simulink model "DAS"  (R2012b)
settings: Solver=FixedStepDiscrete  StartTime=0.0  StopTime=inf  FixedStep=0.1  RelTol=1e-3
PreLoadFcn:
  | if exist('tl_preloadfcn','file'), tl_preloadfcn(gcs,101); end
PostLoadFcn:
  | if exist('tl_postloadfcn','file'), tl_postloadfcn(gcs,101); end
InitFcn:
  | if exist('tlds_init','file'), tlds_init(gcs); end
StartFcn:
  | if exist('tlds_start','file'), tlds_start(gcs); end
StopFcn:
  | if exist('tlds_stop','file'), tlds_stop(gcs); end
undefined symbols (not defined in the file): A, B, C, Dd, DEMO_FAS_Accusti_Threshold_Time, DEMO_FAS_BrakeBooster_Threshold, DEMO_FAS_CC_DELTA, DEMO_FAS_CC_Lvl2_Round, DEMO_FAS_CC_Min_Value, DEMO_FAS_Distance_Treshold_Far, DEMO_FAS_Distance_Treshold_Med, DEMO_FAS_Distance_Treshold_Near, DEMO_FAS_Distronic, DEMO_FAS_Emerg_Brake_Force1, DEMO_FAS_Emerg_Brake_Force2, DEMO_FAS_Emerg_Brake_Time1, DEMO_FAS_Emerg_Brake_Time2, DEMO_FAS_EmergencyBrake, DEMO_FAS_FollowToStop, DEMO_FAS_Limiter, DEMO_FAS_Limiter_DELTA, DEMO_FAS_Neg_Max_ms, DEMO_FAS_Opti_Threshold_Time, DEMO_FAS_Repeater, DEMO_FAS_Repeater_Time, DEMO_FAS_Signdetection, DEMO_FAS_Tempomat
(part 5 of 11)

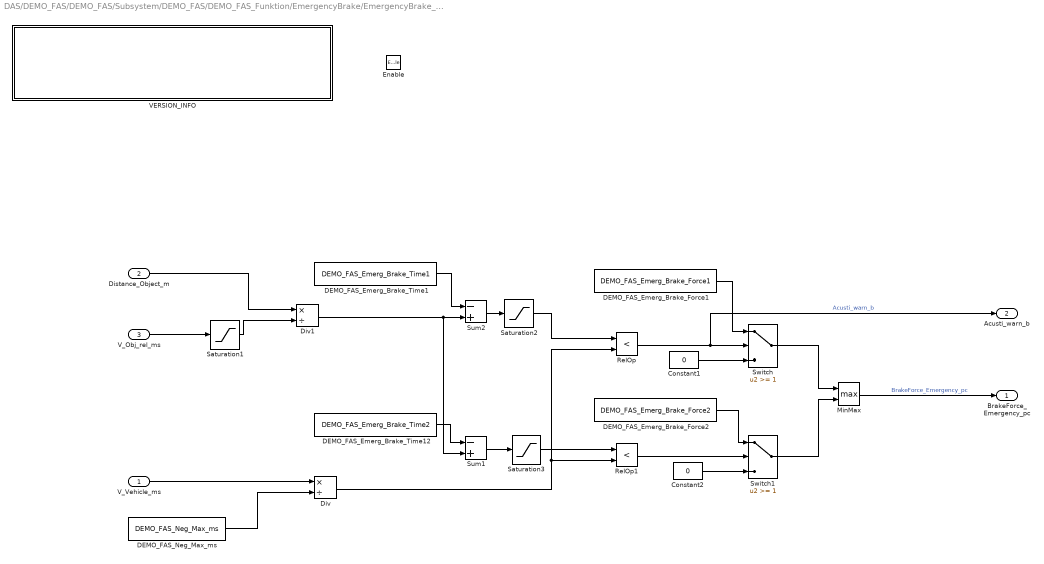
== system DAS/DEMO_FAS/DEMO_FAS/Subsystem/DEMO_FAS/DEMO_FAS_Funktion/EmergencyBrake/EmergencyBrake_Function ==
  V_Vehicle_ms : Inport
  Distance_Object_m : Inport  Port=2
  V_Obj_rel_ms : Inport  Port=3
  Enable : EnablePort  StatesWhenEnabling=reset
  Constant1 : Constant  Value=0  mask(TL_Constant){data={'date',735340.38498962962}}
      settings: CopyFcn=if exist('tl_reset_reviewflag') == 2, tl_reset_reviewflag(gcbh); end  DeleteFcn=if exist('delete_tlblock','file')==2,delete_tlblock(gcbh);end  NameChangeFcn=if exist('rename_tlblock','file')==2,rename_tlblock(gcbh);end  OpenFcn=if exist('tl_open_blockdlg','file')==2,tl_open_blockdlg(gcbh);else,open_system(gcbh,'parameter');end
      mask Help: eval(['if exist(''tl_online_help'',''file'') == 2, tl_online_help(''Topic'',''TL_Constant''),else, web([''jar:file:///'',matlabroot,''/help/toolbox/simulink/help.jar!/slref/' lower(get_param(gcbh,'Blocktype')) '.html''], ''-helpbrowser''),end'])
      mask Display: plot([-0.05, 1.05, NaN, -0.05, 1.05],[.01, .01, NaN, .99, .99])
  Constant2 : Constant  Value=0  mask(TL_Constant){data={'date',735340.38498962962}}
      settings: CopyFcn=if exist('tl_reset_reviewflag') == 2, tl_reset_reviewflag(gcbh); end  DeleteFcn=if exist('delete_tlblock','file')==2,delete_tlblock(gcbh);end  NameChangeFcn=if exist('rename_tlblock','file')==2,rename_tlblock(gcbh);end  OpenFcn=if exist('tl_open_blockdlg','file')==2,tl_open_blockdlg(gcbh);else,open_system(gcbh,'parameter');end
      mask Help: eval(['if exist(''tl_online_help'',''file'') == 2, tl_online_help(''Topic'',''TL_Constant''),else, web([''jar:file:///'',matlabroot,''/help/toolbox/simulink/help.jar!/slref/' lower(get_param(gcbh,'Blocktype')) '.html''], ''-helpbrowser''),end'])
      mask Display: plot([-0.05, 1.05, NaN, -0.05, 1.05],[.01, .01, NaN, .99, .99])
  DEMO_FAS_Emerg_Brake_Force1 : Constant  Description=|  Value=DEMO_FAS_Emerg_Brake_Force1  SampleTime=-1  mask(TL_Constant){data={'output',{'variable','DEMO_FAS/p/Components/DEMO_FAS_Emerg_Brake_Force1'},'date',735389.66854004632}}
      | Constant block of dSPACE TargetLink.
      | 
      | Output signal keeps the given constant value.
      settings: DeleteFcn=if exist('delete_tlblock','file')==2,delete_tlblock(gcbh);end  NameChangeFcn=if exist('rename_tlblock','file')==2,rename_tlblock(gcbh);end  OpenFcn=if exist('tl_open_blockdlg','file')==2,tl_open_blockdlg(gcbh);else,open_system(gcbh,'parameter');end
      mask Help: eval(['if exist(''tl_online_help'',''file'') == 2, tl_online_help(''Topic'',''TL_Constant''),else, web([''jar:file:///'',matlabroot,''/help/toolbox/simulink/help.jar!/slref/' lower(get_param(gcbh,'Blocktype')) '.html''], ''-helpbrowser''),end'])
      mask Display: plot([-0.05, 1.05, NaN, -0.05, 1.05],[.01, .01, NaN, .99, .99])
  DEMO_FAS_Emerg_Brake_Force2 : Constant  Description=|  Value=DEMO_FAS_Emerg_Brake_Force2  SampleTime=-1  mask(TL_Constant){data={'output',{'variable','DEMO_FAS/p/Components/DEMO_FAS_Emerg_Brake_Force2'},'date',735389.66865254624}}
      | Constant block of dSPACE TargetLink.
      | 
      | Output signal keeps the given constant value.
      settings: DeleteFcn=if exist('delete_tlblock','file')==2,delete_tlblock(gcbh);end  NameChangeFcn=if exist('rename_tlblock','file')==2,rename_tlblock(gcbh);end  OpenFcn=if exist('tl_open_blockdlg','file')==2,tl_open_blockdlg(gcbh);else,open_system(gcbh,'parameter');end
      mask Help: eval(['if exist(''tl_online_help'',''file'') == 2, tl_online_help(''Topic'',''TL_Constant''),else, web([''jar:file:///'',matlabroot,''/help/toolbox/simulink/help.jar!/slref/' lower(get_param(gcbh,'Blocktype')) '.html''], ''-helpbrowser''),end'])
      mask Display: plot([-0.05, 1.05, NaN, -0.05, 1.05],[.01, .01, NaN, .99, .99])
  DEMO_FAS_Emerg_Brake_Time1 : Constant  Description=|  Value=DEMO_FAS_Emerg_Brake_Time1  SampleTime=-1  mask(TL_Constant){data={'output',{'variable','DEMO_FAS/p/Components/DEMO_FAS_Emerg_Brake_Time1'},'date',735389.66832118051}}
      | Constant block of dSPACE TargetLink.
      | 
      | Output signal keeps the given constant value.
      settings: DeleteFcn=if exist('delete_tlblock','file')==2,delete_tlblock(gcbh);end  NameChangeFcn=if exist('rename_tlblock','file')==2,rename_tlblock(gcbh);end  OpenFcn=if exist('tl_open_blockdlg','file')==2,tl_open_blockdlg(gcbh);else,open_system(gcbh,'parameter');end
      mask Help: eval(['if exist(''tl_online_help'',''file'') == 2, tl_online_help(''Topic'',''TL_Constant''),else, web([''jar:file:///'',matlabroot,''/help/toolbox/simulink/help.jar!/slref/' lower(get_param(gcbh,'Blocktype')) '.html''], ''-helpbrowser''),end'])
      mask Display: plot([-0.05, 1.05, NaN, -0.05, 1.05],[.01, .01, NaN, .99, .99])
  DEMO_FAS_Emerg_Brake_Time12 : Constant  Description=|  Value=DEMO_FAS_Emerg_Brake_Time2  SampleTime=-1  mask(TL_Constant){data={'output',{'variable','DEMO_FAS/p/Components/DEMO_FAS_Emerg_Brake_Time2'},'date',735389.66844472219}}
      | Constant block of dSPACE TargetLink.
      | 
      | Output signal keeps the given constant value.
      settings: DeleteFcn=if exist('delete_tlblock','file')==2,delete_tlblock(gcbh);end  NameChangeFcn=if exist('rename_tlblock','file')==2,rename_tlblock(gcbh);end  OpenFcn=if exist('tl_open_blockdlg','file')==2,tl_open_blockdlg(gcbh);else,open_system(gcbh,'parameter');end
      mask Help: eval(['if exist(''tl_online_help'',''file'') == 2, tl_online_help(''Topic'',''TL_Constant''),else, web([''jar:file:///'',matlabroot,''/help/toolbox/simulink/help.jar!/slref/' lower(get_param(gcbh,'Blocktype')) '.html''], ''-helpbrowser''),end'])
      mask Display: plot([-0.05, 1.05, NaN, -0.05, 1.05],[.01, .01, NaN, .99, .99])
  DEMO_FAS_Neg_Max_ms : Constant  Description=|  Value=DEMO_FAS_Neg_Max_ms  SampleTime=-1  mask(TL_Constant){data={'output',{'variable','DEMO_FAS/p/Components/DEMO_FAS_Neg_Max_ms'},'date',735389.66875432874}}
      | Constant block of dSPACE TargetLink.
      | 
      | Output signal keeps the given constant value.
      settings: DeleteFcn=if exist('delete_tlblock','file')==2,delete_tlblock(gcbh);end  NameChangeFcn=if exist('rename_tlblock','file')==2,rename_tlblock(gcbh);end  OpenFcn=if exist('tl_open_blockdlg','file')==2,tl_open_blockdlg(gcbh);else,open_system(gcbh,'parameter');end
      mask Help: eval(['if exist(''tl_online_help'',''file'') == 2, tl_online_help(''Topic'',''TL_Constant''),else, web([''jar:file:///'',matlabroot,''/help/toolbox/simulink/help.jar!/slref/' lower(get_param(gcbh,'Blocktype')) '.html''], ''-helpbrowser''),end'])
      mask Display: plot([-0.05, 1.05, NaN, -0.05, 1.05],[.01, .01, NaN, .99, .99])
  Div : Product  Description=|  Inputs=*/  RndMeth=Zero  mask(TL_Product){data={'logdata',{'plotchannels',[]},'date',734383.73388777778}}
      | Product block of dSPACE TargetLink.
      | 
      | Output signal is equal to the product of the input signals. The input ports are specified according to conventions for Simulink Product blocks.
      settings: CopyFcn=if exist('tl_reset_reviewflag') == 2, tl_reset_reviewflag(gcbh); end  DeleteFcn=if exist('delete_tlblock','file')==2,delete_tlblock(gcbh);end  NameChangeFcn=if exist('rename_tlblock','file')==2,rename_tlblock(gcbh);end  OpenFcn=if exist('tl_open_blockdlg','file')==2,tl_open_blockdlg(gcbh);else,open_system(gcbh,'parameter');end
      mask Help: eval(['if exist(''tl_online_help'',''file'') == 2, tl_online_help(''Topic'',''TL_Product''),else, web([''jar:file:///'',matlabroot,''/help/toolbox/simulink/help.jar!/slref/' lower(get_param(gcbh,'Blocktype')) '.html''], ''-helpbrowser''),end'])
      mask Display: plot([-0.05, 1.05, NaN, -0.05, 1.05],[.01, .01, NaN, .99, .99])
  Div1 : Product  Description=|  Inputs=*/  RndMeth=Zero  mask(TL_Product){data={'logdata',{'plotchannels',[]},'date',734383.73388777778}}
      | Product block of dSPACE TargetLink.
      | 
      | Output signal is equal to the product of the input signals. The input ports are specified according to conventions for Simulink Product blocks.
      settings: CopyFcn=if exist('tl_reset_reviewflag') == 2, tl_reset_reviewflag(gcbh); end  DeleteFcn=if exist('delete_tlblock','file')==2,delete_tlblock(gcbh);end  NameChangeFcn=if exist('rename_tlblock','file')==2,rename_tlblock(gcbh);end  OpenFcn=if exist('tl_open_blockdlg','file')==2,tl_open_blockdlg(gcbh);else,open_system(gcbh,'parameter');end
      mask Help: eval(['if exist(''tl_online_help'',''file'') == 2, tl_online_help(''Topic'',''TL_Product''),else, web([''jar:file:///'',matlabroot,''/help/toolbox/simulink/help.jar!/slref/' lower(get_param(gcbh,'Blocktype')) '.html''], ''-helpbrowser''),end'])
      mask Display: plot([-0.05, 1.05, NaN, -0.05, 1.05],[.01, .01, NaN, .99, .99])
  MinMax : MinMax  Description=|  Function=max  Inputs=2  mask(TL_MinMax){data={'logdata',{'plotchannels',[]},'date',735383.52838311344}}
      | MinMax block of dSPACE TargetLink.
      | 
      | The MinMax block outputs either the minimum or the maximum element or elements of the input(s). If the block has one input port, the block outputs a scalar that is the minimum or maximum element of the input vector. If the block has more than one input port, the block performs an element-by-element comparison of the input vectors. Each element of the block output vector is the result of the comparison of the elements of the input vectors. The output of this block is equal to the greater or smaller input depending on the selected function.
      settings: CopyFcn=if exist('tl_reset_reviewflag') == 2, tl_reset_reviewflag(gcbh); end  DeleteFcn=if exist('delete_tlblock','file')==2,delete_tlblock(gcbh);end  NameChangeFcn=if exist('rename_tlblock','file')==2,rename_tlblock(gcbh);end  OpenFcn=if exist('tl_open_blockdlg','file')==2,tl_open_blockdlg(gcbh);else,open_system(gcbh,'parameter');end
      mask Help: eval(['if exist(''tl_online_help'',''file'') == 2, tl_online_help(''Topic'',''TL_MinMax''),else, web([''jar:file:///'',matlabroot,''/help/toolbox/simulink/help.jar!/slref/' lower(get_param(gcbh,'Blocktype')) '.html''], ''-helpbrowser''),end'])
      mask Display: plot([-0.05, 1.05, NaN, -0.05, 1.05],[.01, .01, NaN, .99, .99])
  RelOp : RelationalOperator  Description=|  Operator=<  mask(TL_RelationalOperator){data={'logdata',{'plotchannels',[]},'date',735389.55439398147}}
      | Relational operator block of dSPACE TargetLink.
      | 
      | This block performs a relational operation on its two inputs u1 and u2 and produces output according to the following table.
      | If the result is TRUE, the output is 1; if FALSE, it is 0.
      | 
      | Operator   Output
      |  ==        TRUE if u1 is equal to u2
      |  !=        TRUE if u1 is not equal to u2
      |  <         TRUE if u1 is less than u2
      |  <=        TRUE if u1 is less than or equal to u2
      |  >=        TRUE if u1 is greater than or equal to u2
      |  >         TRUE if u1 is greater than u2
      settings: DeleteFcn=if exist('delete_tlblock','file')==2,delete_tlblock(gcbh);end  NameChangeFcn=if exist('rename_tlblock','file')==2,rename_tlblock(gcbh);end  OpenFcn=if exist('tl_open_blockdlg','file')==2,tl_open_blockdlg(gcbh);else,open_system(gcbh,'parameter');end
      mask Help: eval(['if exist(''tl_online_help'',''file'') == 2, tl_online_help(''Topic'',''TL_RelationalOperator''),else, web([''jar:file:///'',matlabroot,''/help/toolbox/simulink/help.jar!/slref/' lower(get_param(gcbh,'Blocktype')) '.html''], ''-helpbrowser''),end'])
      mask Display: plot([-0.05, 1.05, NaN, -0.05, 1.05],[.01, .01, NaN, .99, .99])
  RelOp1 : RelationalOperator  Description=|  Operator=<  mask(TL_RelationalOperator){data={'logdata',{'plotchannels',[]},'date',735389.55444517359}}
      | Relational operator block of dSPACE TargetLink.
      | 
      | This block performs a relational operation on its two inputs u1 and u2 and produces output according to the following table.
      | If the result is TRUE, the output is 1; if FALSE, it is 0.
      | 
      | Operator   Output
      |  ==        TRUE if u1 is equal to u2
      |  !=        TRUE if u1 is not equal to u2
      |  <         TRUE if u1 is less than u2
      |  <=        TRUE if u1 is less than or equal to u2
      |  >=        TRUE if u1 is greater than or equal to u2
      |  >         TRUE if u1 is greater than u2
      settings: DeleteFcn=if exist('delete_tlblock','file')==2,delete_tlblock(gcbh);end  NameChangeFcn=if exist('rename_tlblock','file')==2,rename_tlblock(gcbh);end  OpenFcn=if exist('tl_open_blockdlg','file')==2,tl_open_blockdlg(gcbh);else,open_system(gcbh,'parameter');end
      mask Help: eval(['if exist(''tl_online_help'',''file'') == 2, tl_online_help(''Topic'',''TL_RelationalOperator''),else, web([''jar:file:///'',matlabroot,''/help/toolbox/simulink/help.jar!/slref/' lower(get_param(gcbh,'Blocktype')) '.html''], ''-helpbrowser''),end'])
      mask Display: plot([-0.05, 1.05, NaN, -0.05, 1.05],[.01, .01, NaN, .99, .99])
  Saturation1 : Saturate  UpperLimit=inf  LowerLimit=1  mask(TL_Saturate){data={'date',735389.55818375002}}
      settings: CopyFcn=if exist('tl_reset_reviewflag') == 2, tl_reset_reviewflag(gcbh); end  DeleteFcn=if exist('delete_tlblock','file')==2,delete_tlblock(gcbh);end  NameChangeFcn=if exist('rename_tlblock','file')==2,rename_tlblock(gcbh);end  OpenFcn=if exist('tl_open_blockdlg','file')==2,tl_open_blockdlg(gcbh);else,open_system(gcbh,'parameter');end
      mask Help: eval(['if exist(''tl_online_help'',''file'') == 2, tl_online_help(''Topic'',''TL_Saturate''),else, web([''jar:file:///'',matlabroot,''/help/toolbox/simulink/help.jar!/slref/' lower(get_param(gcbh,'Blocktype')) '.html''], ''-helpbrowser''),end'])
      mask Display: plot([-0.05, 1.05, NaN, -0.05, 1.05],[.01, .01, NaN, .99, .99])
  Saturation2 : Saturate  UpperLimit=inf  LowerLimit=1  mask(TL_Saturate){data={'date',735389.55818375002}}
      settings: CopyFcn=if exist('tl_reset_reviewflag') == 2, tl_reset_reviewflag(gcbh); end  DeleteFcn=if exist('delete_tlblock','file')==2,delete_tlblock(gcbh);end  NameChangeFcn=if exist('rename_tlblock','file')==2,rename_tlblock(gcbh);end  OpenFcn=if exist('tl_open_blockdlg','file')==2,tl_open_blockdlg(gcbh);else,open_system(gcbh,'parameter');end
      mask Help: eval(['if exist(''tl_online_help'',''file'') == 2, tl_online_help(''Topic'',''TL_Saturate''),else, web([''jar:file:///'',matlabroot,''/help/toolbox/simulink/help.jar!/slref/' lower(get_param(gcbh,'Blocktype')) '.html''], ''-helpbrowser''),end'])
      mask Display: plot([-0.05, 1.05, NaN, -0.05, 1.05],[.01, .01, NaN, .99, .99])
  Saturation3 : Saturate  UpperLimit=inf  LowerLimit=1  mask(TL_Saturate){data={'date',735389.55818375002}}
      settings: CopyFcn=if exist('tl_reset_reviewflag') == 2, tl_reset_reviewflag(gcbh); end  DeleteFcn=if exist('delete_tlblock','file')==2,delete_tlblock(gcbh);end  NameChangeFcn=if exist('rename_tlblock','file')==2,rename_tlblock(gcbh);end  OpenFcn=if exist('tl_open_blockdlg','file')==2,tl_open_blockdlg(gcbh);else,open_system(gcbh,'parameter');end
      mask Help: eval(['if exist(''tl_online_help'',''file'') == 2, tl_online_help(''Topic'',''TL_Saturate''),else, web([''jar:file:///'',matlabroot,''/help/toolbox/simulink/help.jar!/slref/' lower(get_param(gcbh,'Blocktype')) '.html''], ''-helpbrowser''),end'])
      mask Display: plot([-0.05, 1.05, NaN, -0.05, 1.05],[.01, .01, NaN, .99, .99])
  Sum1 : Sum  Description=|  Inputs=-+  mask(TL_Sum){data={'logdata',{'plotchannels',[]},'date',735383.47236888891}}
      | Sum block of dSPACE TargetLink.
      | 
      | Output signal is equal to the sum of the input signals.
      | The list of signs is specified according to conventions for Simulink Sum blocks.
      settings: CopyFcn=if exist('tl_reset_reviewflag') == 2, tl_reset_reviewflag(gcbh); end  DeleteFcn=if exist('delete_tlblock','file')==2,delete_tlblock(gcbh);end  NameChangeFcn=if exist('rename_tlblock','file')==2,rename_tlblock(gcbh);end  OpenFcn=if exist('tl_open_blockdlg','file')==2,tl_open_blockdlg(gcbh);else,open_system(gcbh,'parameter');end
      mask Help: eval(['if exist(''tl_online_help'',''file'') == 2, tl_online_help(''Topic'',''TL_Sum''),else, web([''jar:file:///'',matlabroot,''/help/toolbox/simulink/help.jar!/slref/' lower(get_param(gcbh,'Blocktype')) '.html''], ''-helpbrowser''),end'])
      mask Display: plot([-0.05, 1.05, NaN, -0.05, 1.05],[.01, .01, NaN, .99, .99])
  Sum2 : Sum  Description=|  Inputs=-+  mask(TL_Sum){data={'logdata',{'plotchannels',[]},'date',735383.47236888891}}
      | Sum block of dSPACE TargetLink.
      | 
      | Output signal is equal to the sum of the input signals.
      | The list of signs is specified according to conventions for Simulink Sum blocks.
      settings: CopyFcn=if exist('tl_reset_reviewflag') == 2, tl_reset_reviewflag(gcbh); end  DeleteFcn=if exist('delete_tlblock','file')==2,delete_tlblock(gcbh);end  NameChangeFcn=if exist('rename_tlblock','file')==2,rename_tlblock(gcbh);end  OpenFcn=if exist('tl_open_blockdlg','file')==2,tl_open_blockdlg(gcbh);else,open_system(gcbh,'parameter');end
      mask Help: eval(['if exist(''tl_online_help'',''file'') == 2, tl_online_help(''Topic'',''TL_Sum''),else, web([''jar:file:///'',matlabroot,''/help/toolbox/simulink/help.jar!/slref/' lower(get_param(gcbh,'Blocktype')) '.html''], ''-helpbrowser''),end'])
      mask Display: plot([-0.05, 1.05, NaN, -0.05, 1.05],[.01, .01, NaN, .99, .99])
  Switch : Switch  Threshold=1  mask(TL_Switch){data={'date',735389.55168915505}}
      settings: CopyFcn=if exist('tl_reset_reviewflag') == 2, tl_reset_reviewflag(gcbh); end  DeleteFcn=if exist('delete_tlblock','file')==2,delete_tlblock(gcbh);end  NameChangeFcn=if exist('rename_tlblock','file')==2,rename_tlblock(gcbh);end  OpenFcn=if exist('tl_open_blockdlg','file')==2,tl_open_blockdlg(gcbh);else,open_system(gcbh,'parameter');end
      mask Help: eval(['if exist(''tl_online_help'',''file'') == 2, tl_online_help(''Topic'',''TL_Switch''),else, web([''jar:file:///'',matlabroot,''/help/toolbox/simulink/help.jar!/slref/' lower(get_param(gcbh,'Blocktype')) '.html''], ''-helpbrowser''),end'])
      mask Display: plot([-0.05, 1.05, NaN, -0.05, 1.05],[.01, .01, NaN, .99, .99])
  Switch1 : Switch  Threshold=1  mask(TL_Switch){data={'date',735383.52020709496}}
      settings: CopyFcn=if exist('tl_reset_reviewflag') == 2, tl_reset_reviewflag(gcbh); end  DeleteFcn=if exist('delete_tlblock','file')==2,delete_tlblock(gcbh);end  NameChangeFcn=if exist('rename_tlblock','file')==2,rename_tlblock(gcbh);end  OpenFcn=if exist('tl_open_blockdlg','file')==2,tl_open_blockdlg(gcbh);else,open_system(gcbh,'parameter');end
      mask Help: eval(['if exist(''tl_online_help'',''file'') == 2, tl_online_help(''Topic'',''TL_Switch''),else, web([''jar:file:///'',matlabroot,''/help/toolbox/simulink/help.jar!/slref/' lower(get_param(gcbh,'Blocktype')) '.html''], ''-helpbrowser''),end'])
      mask Display: plot([-0.05, 1.05, NaN, -0.05, 1.05],[.01, .01, NaN, .99, .99])
  VERSION_INFO : Subsystem  mask(VERSION_INFO_BLOCK){versinfo_data=struct('modname','DEMO_FAS/DEMO_FAS_Funktion/EmergencyBrake/EmergencyBrake_Function','version','1.1.1','date','29-May-2013','author','YVEDUHR','modtype',3,'variant',0,'remark',{{'~'}},'copyright',['Daimler AG'],'SGMLdescr','','prefix','','pfx_act',0,'ntselect',3,'asize',0), versinfo_string=Model: DEMO_FAS/DEMO_FAS_Funktion/EmergencyBrake/EmergencyBrake_Function\nVersion: 1.1.1\nDate: 29-May-2013\nAuthor: YVEDUHR\nModule: INTERNAL\n\nAll copyrights by Daimler AG}
      mask prompts: versinfo_data "Mask Parameter 1"; versinfo_string "Mask Parameter 2"
      mask help:
      | This is a Version Info Subsystem (empty)
      | All version Information is stored in Parameter "versinfo_data" and displayed
      settings: OpenFcn=edit_subsys_info('init')
      mask Display: disp(versinfo_string);
  BrakeForce_Emergency_pc : Outport  InitialOutput=0
  Acusti_warn_b : Outport  Port=2  InitialOutput=0
  wires:
  V_Vehicle_ms/1 -> Div/1
  DEMO_FAS_Neg_Max_ms/1 -> Div/2
  Div/1 -> RelOp/2, RelOp1/2
  Distance_Object_m/1 -> Div1/1
  V_Obj_rel_ms/1 -> Saturation1/1
  DEMO_FAS_Emerg_Brake_Time1/1 -> Sum2/1
  DEMO_FAS_Emerg_Brake_Time12/1 -> Sum1/1
  Sum2/1 -> Saturation2/1
  Sum1/1 -> Saturation3/1
  RelOp/1 -> Acusti_warn_b/1, Switch/2  "Acusti_warn_b"
  DEMO_FAS_Emerg_Brake_Force1/1 -> Switch/1
  DEMO_FAS_Emerg_Brake_Force2/1 -> Switch1/1
  RelOp1/1 -> Switch1/2
  Constant1/1 -> Switch/3
  Constant2/1 -> Switch1/3
  Switch/1 -> MinMax/1
  Switch1/1 -> MinMax/2
  MinMax/1 -> BrakeForce_Emergency_pc/1  "BrakeForce_Emergency_pc"
  Div1/1 -> Sum1/2, Sum2/2
  Saturation1/1 -> Div1/2
  Saturation2/1 -> RelOp/1
  Saturation3/1 -> RelOp1/1

== system DAS/DEMO_FAS/DEMO_FAS/Subsystem/DEMO_FAS/DEMO_FAS_Funktion/EmergencyBrake/VERSION_INFO ==
  Copyright : Subsystem
      mask help: Copyright
      mask Display: disp('All copyrights by DaimlerChrysler');

== system DAS/DEMO_FAS/DEMO_FAS/Subsystem/DEMO_FAS/DEMO_FAS_Funktion/FAS_Input/VERSION_INFO ==
  Copyright : Subsystem
      mask help: Copyright
      mask Display: disp('All copyrights by DaimlerChrysler');

== system DAS/DEMO_FAS/DEMO_FAS/Subsystem/DEMO_FAS/DEMO_FAS_Funktion/FollowToStop/FollowToStop_Function ==
  V_Vehicle_kmh : Inport
  V_Obj_rel_kmh : Inport  Port=2
  Enable : EnablePort  StatesWhenEnabling=reset
  Chart : Stateflow chart  TreatAsAtomicUnit=on
  Sum : Sum  Description=|  Inputs=+-  mask(TL_Sum){data={'logdata',{'plotchannels',[]},'date',735388.57141554402}}
      | Sum block of dSPACE TargetLink.
      | 
      | Output signal is equal to the sum of the input signals.
      | The list of signs is specified according to conventions for Simulink Sum blocks.
      settings: CopyFcn=if exist('tl_reset_reviewflag') == 2, tl_reset_reviewflag(gcbh); end  DeleteFcn=if exist('delete_tlblock','file')==2,delete_tlblock(gcbh);end  NameChangeFcn=if exist('rename_tlblock','file')==2,rename_tlblock(gcbh);end  OpenFcn=if exist('tl_open_blockdlg','file')==2,tl_open_blockdlg(gcbh);else,open_system(gcbh,'parameter');end
      mask Help: eval(['if exist(''tl_online_help'',''file'') == 2, tl_online_help(''Topic'',''TL_Sum''),else, web([''jar:file:///'',matlabroot,''/help/toolbox/simulink/help.jar!/slref/' lower(get_param(gcbh,'Blocktype')) '.html''], ''-helpbrowser''),end'])
      mask Display: plot([-0.05, 1.05, NaN, -0.05, 1.05],[.01, .01, NaN, .99, .99])
  VERSION_INFO : Subsystem  mask(VERSION_INFO_BLOCK){versinfo_data=struct('modname','DEMO_FAS/DEMO_FAS_Funktion/FollowToStop/FollowToStop_Function','version','1.1.1','date','23-May-2013','author','YVEDUHR','modtype',3,'variant',0,'remark',{{'~'}},'copyright',['Daimler AG'],'SGMLdescr','','prefix','','pfx_act',0,'ntselect',3,'asize',0), versinfo_string=Model: DEMO_FAS/DEMO_FAS_Funktion/FollowToStop/FollowToStop_Function\nVersion: 1.1.1\nDate: 23-May-2013\nAuthor: YVEDUHR\nModule: INTERNAL\n\nAll copyrights by Daimler AG}
      mask prompts: versinfo_data "Mask Parameter 1"; versinfo_string "Mask Parameter 2"
      mask help:
      | This is a Version Info Subsystem (empty)
      | All version Information is stored in Parameter "versinfo_data" and displayed
      settings: OpenFcn=edit_subsys_info('init')
      mask Display: disp(versinfo_string);
  FTS_active_b : Outport
  FTS_Abstand_soll_m : Outport  Port=2
  wires:
  V_Obj_rel_kmh/1 -> Sum/2
  V_Vehicle_kmh/1 -> Sum/1
  Sum/1 -> Chart/1(V_Obj_kmh)  "V_Obj_kmh"
  Chart/1(FTS_active_b) -> FTS_active_b/1  "FTS_active_b"
  Chart/2(Abstand_soll_m) -> FTS_Abstand_soll_m/1  "FTS_Abstand_soll_m"

== system DAS/DEMO_FAS/DEMO_FAS/Subsystem/DEMO_FAS/DEMO_FAS_Funktion/FollowToStop/VERSION_INFO ==
  Copyright : Subsystem
      mask help: Copyright
      mask Display: disp('All copyrights by DaimlerChrysler');

== system DAS/DEMO_FAS/DEMO_FAS/Subsystem/DEMO_FAS/DEMO_FAS_Funktion/Limiter/Limiter_Function ==
  Limiter_b : Inport
  Accelaration_pedal_pc : Inport  Port=2
  V_Vehicle_kmh : Inport  Port=3
  LeverUp_stat : Inport  Port=4
  LeverDown_stat : Inport  Port=5
  V_Sign_kmh : Inport  Port=6
  Sign_b : Inport  Port=7
  Enable : EnablePort
  DEMO_FAS_Signdetection : Constant  Description=|  Value=DEMO_FAS_Signdetection  SampleTime=-1  mask(TL_Constant){data={'output',{'variable','DEMO_FAS/p/Components/DEMO_FAS_Signdetection'},'date',735441.46049939818}}
      | Constant block of dSPACE TargetLink.
      | 
      | Output signal keeps the given constant value.
      settings: DeleteFcn=if exist('delete_tlblock','file')==2,delete_tlblock(gcbh);end  NameChangeFcn=if exist('rename_tlblock','file')==2,rename_tlblock(gcbh);end  OpenFcn=if exist('tl_open_blockdlg','file')==2,tl_open_blockdlg(gcbh);else,open_system(gcbh,'parameter');end
      mask Help: eval(['if exist(''tl_online_help'',''file'') == 2, tl_online_help(''Topic'',''TL_Constant''),else, web([''jar:file:///'',matlabroot,''/help/toolbox/simulink/help.jar!/slref/' lower(get_param(gcbh,'Blocktype')) '.html''], ''-helpbrowser''),end'])
      mask Display: plot([-0.05, 1.05, NaN, -0.05, 1.05],[.01, .01, NaN, .99, .99])
  Limiter_Enabled : Subsystem
  Limiter_InitialSetValue : Subsystem  TreatAsAtomicUnit=on
  Limiter_SetValue : Subsystem
  Limiter_StartUpSetValue : Subsystem  TreatAsAtomicUnit=on
  Logical Operator : Logic  AllPortsSameDT=off  OutDataTypeStr=boolean  mask(TL_LogicalOperator){data={'date',735360.45292877313}}
      settings: DeleteFcn=if exist('delete_tlblock','file')==2,delete_tlblock(gcbh);end  NameChangeFcn=if exist('rename_tlblock','file')==2,rename_tlblock(gcbh);end  OpenFcn=if exist('tl_open_blockdlg','file')==2,tl_open_blockdlg(gcbh);else,open_system(gcbh,'parameter');end
      mask Help: eval(['if exist(''tl_online_help'',''file'') == 2, tl_online_help(''Topic'',''TL_LogicalOperator''),else, web([''jar:file:///'',matlabroot,''/help/toolbox/simulink/help.jar!/slref/' lower(get_param(gcbh,'Blocktype')) '.html''], ''-helpbrowser''),end'])
      mask Display: plot([-0.05, 1.05, NaN, -0.05, 1.05],[.01, .01, NaN, .99, .99])
  MinMax : MinMax  Inputs=2  mask(TL_MinMax){data={'date',735369.40750826395}}
      settings: CopyFcn=if exist('tl_reset_reviewflag') == 2, tl_reset_reviewflag(gcbh); end  DeleteFcn=if exist('delete_tlblock','file')==2,delete_tlblock(gcbh);end  NameChangeFcn=if exist('rename_tlblock','file')==2,rename_tlblock(gcbh);end  OpenFcn=if exist('tl_open_blockdlg','file')==2,tl_open_blockdlg(gcbh);else,open_system(gcbh,'parameter');end
      mask Help: eval(['if exist(''tl_online_help'',''file'') == 2, tl_online_help(''Topic'',''TL_MinMax''),else, web([''jar:file:///'',matlabroot,''/help/toolbox/simulink/help.jar!/slref/' lower(get_param(gcbh,'Blocktype')) '.html''], ''-helpbrowser''),end'])
      mask Display: plot([-0.05, 1.05, NaN, -0.05, 1.05],[.01, .01, NaN, .99, .99])
  Switch : Switch  Threshold=1  mask(TL_Switch){data={'date',735369.40809475689}}
      settings: CopyFcn=if exist('tl_reset_reviewflag') == 2, tl_reset_reviewflag(gcbh); end  DeleteFcn=if exist('delete_tlblock','file')==2,delete_tlblock(gcbh);end  NameChangeFcn=if exist('rename_tlblock','file')==2,rename_tlblock(gcbh);end  OpenFcn=if exist('tl_open_blockdlg','file')==2,tl_open_blockdlg(gcbh);else,open_system(gcbh,'parameter');end
      mask Help: eval(['if exist(''tl_online_help'',''file'') == 2, tl_online_help(''Topic'',''TL_Switch''),else, web([''jar:file:///'',matlabroot,''/help/toolbox/simulink/help.jar!/slref/' lower(get_param(gcbh,'Blocktype')) '.html''], ''-helpbrowser''),end'])
      mask Display: plot([-0.05, 1.05, NaN, -0.05, 1.05],[.01, .01, NaN, .99, .99])
  SysInit : Subsystem  mask(TLACT_SG_V200_SysInit){dT=-1, YName=}
      mask prompts: dT "Sample Time"; YName "Y OutName"
      mask help: An inital pulse is generated for for the first block evaluation.
      mask init:
      | % TL block lines
      | x1=[0 0 1 1 0];
      | y1=[1 0 0 1 1];
      | x2=[1 0];
      | y2=[.92 .92];
      | x3=[0 1];
      | y3=[.08 .08];
      | 
      | tl_act_sg_init_blk;
      mask Help:
      | <P><B>Function:</B></P>
      | <P>The block provides an initial pulse at the output on the first
      | evaluation of the block.<BR> This function can be used for system startup functions to
      | get defined states in the system.</P>
      | 
      | <P><B>In-/Outputs:</B></P>
      | <P><U>Output</U></P>
      | <P>The output shows TRUE at the first cycle, else it shows FALSE.</P>
      mask Display:
      | plot(x1,y1,x2,y2,x3,y3);
      | disp('SysInit');
  VERSION_INFO : Subsystem  mask(VERSION_INFO_BLOCK){versinfo_data=struct('modname','DEMO_FAS/DEMO_FAS_Funktion/Limiter/Limiter_Function','version','1.1.1','date','18-Apr-2013','author','YVEDUHR','modtype',3,'variant',0,'remark',{{'~'}},'copyright',['Daimler AG'],'SGMLdescr','','prefix','','pfx_act',0,'ntselect',3,'asize',0), versinfo_string=Model: DEMO_FAS/DEMO_FAS_Funktion/Limiter/Limiter_Function\nVersion: 1.1.1\nDate: 18-Apr-2013\nAuthor: YVEDUHR\nModule: INTERNAL\n\nAll copyrights by Daimler AG}
      mask prompts: versinfo_data "Mask Parameter 1"; versinfo_string "Mask Parameter 2"
      mask help:
      | This is a Version Info Subsystem (empty)
      | All version Information is stored in Parameter "versinfo_data" and displayed
      settings: OpenFcn=edit_subsys_info('init')
      mask Display: disp(versinfo_string);
  VMax_kmh : Outport
  Limiter_active_b : Outport  Port=2  InitialOutput=0
  wires:
  LeverDown_stat/1 -> Limiter_SetValue/2(LeverDown_stat)
  LeverUp_stat/1 -> Limiter_SetValue/1(LeverUp_stat)
  V_Vehicle_kmh/1 -> Limiter_InitialSetValue/1(V_Vehicle_kmh)
  Limiter_Enabled/1(VMax_kmh) -> MinMax/2, Switch/3
  Limiter_b/1 -> Limiter_InitialSetValue/Trigger, Limiter_SetValue/Enable, Limiter_Enabled/1(Limiter_b)
  Accelaration_pedal_pc/1 -> Limiter_Enabled/2(Accelaration_pedal_pc)
  Limiter_Enabled/2(Limiter_active_b) -> Limiter_active_b/1
  SysInit/1(y) -> Limiter_StartUpSetValue/Trigger
  Switch/1 -> VMax_kmh/1  "VMax_kmh"
  Sign_b/1 -> Logical Operator/1
  MinMax/1 -> Switch/1
  V_Sign_kmh/1 -> MinMax/1
  DEMO_FAS_Signdetection/1 -> Logical Operator/2
  Logical Operator/1 -> Switch/2

== system DAS/DEMO_FAS/DEMO_FAS/Subsystem/DEMO_FAS/DEMO_FAS_Funktion/Limiter/VERSION_INFO ==
  Copyright : Subsystem
      mask help: Copyright
      mask Display: disp('All copyrights by DaimlerChrysler');

== system DAS/DEMO_FAS/DEMO_FAS/Subsystem/DEMO_FAS/DEMO_FAS_Funktion/Tempomat/Tempomat_Function ==
  ParkingBrake_b : Inport
  BrakeForce_pedal_pc : Inport  Port=2
  CruiseControl_b : Inport  Port=3
  V_Vehicle_kmh : Inport  Port=4
  Limiter_b : Inport  Port=5
  LeverUp_Stat : Inport  Port=6
  LeverDown_Stat : Inport  Port=7
  FTS_active_b : Inport  Port=8
  Enable : EnablePort
  CC_Enabled : Subsystem
  CC_On_Off : Subsystem
  CC_SetValue : Subsystem
  VERSION_INFO : Subsystem  mask(VERSION_INFO_BLOCK){versinfo_data=struct('modname','DEMO_FAS/DEMO_FAS_Funktion/Tempomat/Tempomat_Function','version','1.1.1','date','19-Apr-2013','author','YVEDUHR','modtype',3,'variant',0,'remark',{{'~'}},'copyright',['Daimler AG'],'SGMLdescr','','prefix','','pfx_act',0,'ntselect',3,'asize',0), versinfo_string=Model: DEMO_FAS/DEMO_FAS_Funktion/Tempomat/Tempomat_Function\nVersion: 1.1.1\nDate: 19-Apr-2013\nAuthor: YVEDUHR\nModule: INTERNAL\n\nAll copyrights by Daimler AG}
      mask prompts: versinfo_data "Mask Parameter 1"; versinfo_string "Mask Parameter 2"
      mask help:
      | This is a Version Info Subsystem (empty)
      | All version Information is stored in Parameter "versinfo_data" and displayed
      settings: OpenFcn=edit_subsys_info('init')
      mask Display: disp(versinfo_string);
  V_CC_delta_kmh : Outport  OutputWhenDisabled=reset  InitialOutput=0
  CC_active_b : Outport  Port=2  OutputWhenDisabled=reset  InitialOutput=0
  wires:
  LeverDown_Stat/1 -> CC_On_Off/7(LeverDown_stat), CC_SetValue/6(LeverDown_Stat)
  LeverUp_Stat/1 -> CC_On_Off/6(LeverUp_stat), CC_SetValue/5(LeverUp_Stat)
  CC_Enabled/1(V_CC_delta_kmh) -> V_CC_delta_kmh/1
  V_Vehicle_kmh/1 -> CC_On_Off/4(V_Vehicle_kmh), CC_SetValue/4(V_Vehicle_kmh), CC_Enabled/2(V_Vehicle_kmh)
  CruiseControl_b/1 -> CC_SetValue/3(CruiseControl_b), CC_On_Off/3(CruiseControl_b)
  ParkingBrake_b/1 -> CC_On_Off/1(ParkingBrake_b)
  BrakeForce_pedal_pc/1 -> CC_On_Off/2(BrakeForce_pedal_pc)
  CC_On_Off/1(CC_active_b) -> CC_active_b/1, CC_SetValue/2(CC_enabled_b), CC_Enabled/1(CC_active_b)
  Limiter_b/1 -> CC_SetValue/1(Limiter_b), CC_On_Off/5(Limiter_b)
  FTS_active_b/1 -> CC_On_Off/8(FTS_active_b)

== system DAS/DEMO_FAS/DEMO_FAS/Subsystem/DEMO_FAS/DEMO_FAS_Funktion/Tempomat/VERSION_INFO ==
  Copyright : Subsystem
      mask help: Copyright
      mask Display: disp('All copyrights by DaimlerChrysler');

== system DAS/DEMO_FAS/DEMO_FAS/Subsystem/DEMO_FAS/DEMO_FAS_Funktion/VERSION_INFO/Copyright ==

== system DAS/DEMO_FAS/DEMO_FAS/Subsystem/DEMO_FAS/DEMO_FAS_Funktion/Velocity Control/VERSION_INFO ==
  Copyright : Subsystem
      mask help: Copyright
      mask Display: disp('All copyrights by DaimlerChrysler');

== system DAS/DEMO_FAS/DEMO_FAS/Subsystem/DEMO_FAS/DEMO_FAS_Funktion/BrakeAssistant/Brake_Booster/VERSION_INFO ==
  Copyright : Subsystem
      mask help: Copyright
      mask Display: disp('All copyrights by DaimlerChrysler');

== system DAS/DEMO_FAS/DEMO_FAS/Subsystem/DEMO_FAS/DEMO_FAS_Funktion/BrakeAssistant/VERSION_INFO/Copyright ==

== system DAS/DEMO_FAS/DEMO_FAS/Subsystem/DEMO_FAS/DEMO_FAS_Funktion/Distancewarner/Distancewarner_Function/VERSION_INFO ==
  Copyright : Subsystem
      mask help: Copyright
      mask Display: disp('All copyrights by DaimlerChrysler');

== system DAS/DEMO_FAS/DEMO_FAS/Subsystem/DEMO_FAS/DEMO_FAS_Funktion/Distancewarner/VERSION_INFO/Copyright ==

== system DAS/DEMO_FAS/DEMO_FAS/Subsystem/DEMO_FAS/DEMO_FAS_Funktion/Distronic/Distronic_Deactive/VERSION_INFO ==
  Copyright : Subsystem
      mask help: Copyright
      mask Display: disp('All copyrights by DaimlerChrysler');

== system DAS/DEMO_FAS/DEMO_FAS/Subsystem/DEMO_FAS/DEMO_FAS_Funktion/Distronic/Distronic_Disabled/VERSION_INFO ==
  Copyright : Subsystem
      mask help: Copyright
      mask Display: disp('All copyrights by DaimlerChrysler');

== system DAS/DEMO_FAS/DEMO_FAS/Subsystem/DEMO_FAS/DEMO_FAS_Funktion/Distronic/Distronic_Enabled/VERSION_INFO ==
  Copyright : Subsystem
      mask help: Copyright
      mask Display: disp('All copyrights by DaimlerChrysler');

== system DAS/DEMO_FAS/DEMO_FAS/Subsystem/DEMO_FAS/DEMO_FAS_Funktion/Distronic/Distronic_FTS_Enabled/VERSION_INFO ==
  Copyright : Subsystem
      mask help: Copyright
      mask Display: disp('All copyrights by DaimlerChrysler');

== system DAS/DEMO_FAS/DEMO_FAS/Subsystem/DEMO_FAS/DEMO_FAS_Funktion/Distronic/VERSION_INFO/Copyright ==

== system DAS/DEMO_FAS/DEMO_FAS/Subsystem/DEMO_FAS/DEMO_FAS_Funktion/EmergencyBrake/EmergencyBrake_Function/VERSION_INFO ==
  Copyright : Subsystem
      mask help: Copyright
      mask Display: disp('All copyrights by DaimlerChrysler');

== system DAS/DEMO_FAS/DEMO_FAS/Subsystem/DEMO_FAS/DEMO_FAS_Funktion/EmergencyBrake/VERSION_INFO/Copyright ==

== system DAS/DEMO_FAS/DEMO_FAS/Subsystem/DEMO_FAS/DEMO_FAS_Funktion/FAS_Input/VERSION_INFO/Copyright ==

== system DAS/DEMO_FAS/DEMO_FAS/Subsystem/DEMO_FAS/DEMO_FAS_Funktion/FollowToStop/FollowToStop_Function/VERSION_INFO ==
  Copyright : Subsystem
      mask help: Copyright
      mask Display: disp('All copyrights by DaimlerChrysler');

== system DAS/DEMO_FAS/DEMO_FAS/Subsystem/DEMO_FAS/DEMO_FAS_Funktion/FollowToStop/VERSION_INFO/Copyright ==

== system DAS/DEMO_FAS/DEMO_FAS/Subsystem/DEMO_FAS/DEMO_FAS_Funktion/Limiter/Limiter_Function/Limiter_Enabled ==
  Limiter_b : Inport
  Accelaration_pedal_pc : Inport  Port=2
  Bus Creator : BusCreator  Inputs=2
  Bus Creator1 : BusCreator  Inputs=2
  Bus Selector : BusSelector  OutputSignals=VMax_kmh,Limiter_active_b
  EdgeRising : Subsystem  mask(TLMSR_V200_EdgeRising){dT=-1, YName=}
      mask prompts: dT "Sampe Time"; YName "Y OutName"
      mask help:
      | The output indicates TRUE if the input value changes from FALSE to TRUE.
      | Reset input 'R' on TRUE will write the initial value 'IV' to the internal memory.
      mask init:
      | % TL block lines
      | x1=[0 0 1 1 0];
      | y1=[1 0 0 1 1];
      | x2=[1 0];
      | y2=[.96 .96];
      | x3=[0 1];
      | y3=[.04 .04];
      | 
      | tl_act_sg_init_blk;
      mask Help:
      | <HTML>
      | <HEAD>
      | <META HTTP-EQUIV="Content-Type" CONTENT="text/html; charset=iso-8859-1">
      | <TITLE>Help</TITLE>
      | </HEAD>
      | <BODY>
      | 
      | <B><FONT FACE="Arial"><P>Function:</P>
      | </B><P>The block detects a rising edge of the logical input signal <FONT FACE="Courier New">u</FONT> and indicates this change at the output <FONT FACE="Courier New">y</FONT> for one cycle.</P>
      | 
      | <B><P>In-/Outputs:</P>
      | </B>
      | <P><U>Input</U></P>
      | <P>The block input </FONT><FONT FACE="Courier New">u</FONT><FONT FACE="Arial"> must be connected to the input signal.</P>
      | 
      | <U><P>Reset / Initial Value</P>
      | </U><P>If the reset input </FONT><FONT FACE="Courier New">R</FONT><FONT FACE="Arial"> gets a '1' signal the block will write the initial value <FONT FACE="Courier New">IV</FONT> to its internal memory. A logical '1' at <FONT FACE="Courier New">IV</FONT>
      | will prevent the output to become TRUE during reset.</P>
      | 
      | <U><P>Output</P>
      | </U><P>The output </FONT><FONT FACE="Courier New">y</FONT><FONT FACE="Arial"> shows '1' if a rising edge at the input signal <FONT FACE="Courier New">u</FONT> is detected.</P>
      | </FONT></BODY>
      | </HTML>
      mask Display:
      | plot(x1,y1,x2,y2,x3,y3);
      | image(imread('EdgeRising.tif','tif'),[0.25,0.2,0.5,0.6])
  False : Subsystem  mask(TLACT_SG_V200_False){}
      mask help: False
      mask init:
      | % TL block lines
      | x1=[0 0 1 1 0];
      | y1=[1 0 0 1 1];
      | x2=[1 0];
      | y2=[.9 .9];
      | x3=[0 1];
      | y3=[.1 .1];
      settings: OpenFcn=open_system([gcb, '/Zero'], 'OpenFcn')
      mask Display:
      | plot(x1,y1,x2,y2,x3,y3);
      | disp('False');
  If : If  NumInputs=2  IfExpression=u2 & u1 < 90
  Limiter_Active : Subsystem  TreatAsAtomicUnit=on
  Limiter_Deactive : Subsystem  TreatAsAtomicUnit=on
  Logical Operator1 : Logic  Operator=NOT  Inputs=1  AllPortsSameDT=off  OutDataTypeStr=boolean  mask(TL_LogicalOperator){data={'date',735339.71002042829}}
      settings: DeleteFcn=if exist('delete_tlblock','file')==2,delete_tlblock(gcbh);end  NameChangeFcn=if exist('rename_tlblock','file')==2,rename_tlblock(gcbh);end  OpenFcn=if exist('tl_open_blockdlg','file')==2,tl_open_blockdlg(gcbh);else,open_system(gcbh,'parameter');end
      mask Help: eval(['if exist(''tl_online_help'',''file'') == 2, tl_online_help(''Topic'',''TL_LogicalOperator''),else, web([''jar:file:///'',matlabroot,''/help/toolbox/simulink/help.jar!/slref/' lower(get_param(gcbh,'Blocktype')) '.html''], ''-helpbrowser''),end'])
      mask Display: plot([-0.05, 1.05, NaN, -0.05, 1.05],[.01, .01, NaN, .99, .99])
  Logical Operator2 : Logic  Operator=NOT  Inputs=1  AllPortsSameDT=off  OutDataTypeStr=boolean  mask(TL_LogicalOperator){data={'date',735339.71002042829}}
      settings: DeleteFcn=if exist('delete_tlblock','file')==2,delete_tlblock(gcbh);end  NameChangeFcn=if exist('rename_tlblock','file')==2,rename_tlblock(gcbh);end  OpenFcn=if exist('tl_open_blockdlg','file')==2,tl_open_blockdlg(gcbh);else,open_system(gcbh,'parameter');end
      mask Help: eval(['if exist(''tl_online_help'',''file'') == 2, tl_online_help(''Topic'',''TL_LogicalOperator''),else, web([''jar:file:///'',matlabroot,''/help/toolbox/simulink/help.jar!/slref/' lower(get_param(gcbh,'Blocktype')) '.html''], ''-helpbrowser''),end'])
      mask Display: plot([-0.05, 1.05, NaN, -0.05, 1.05],[.01, .01, NaN, .99, .99])
  Merge : Merge  Description=|  mask(TL_Merge){data={'date',735441.37729406252}}
      | Merge block of dSPACE TargetLink.
      | 
      | Use this block instead of Simulink's Merge block if you wish to control how merge variables should be generated.
      settings: CopyFcn=if exist('tl_reset_reviewflag') == 2, tl_reset_reviewflag(gcbh); end  DeleteFcn=if exist('delete_tlblock','file')==2,delete_tlblock(gcbh);end  NameChangeFcn=if exist('rename_tlblock','file')==2,rename_tlblock(gcbh);end  OpenFcn=if exist('tl_open_blockdlg','file')==2,tl_open_blockdlg(gcbh);else,open_system(gcbh,'parameter');end
      mask Help: eval(['if exist(''tl_online_help'',''file'') == 2, tl_online_help(''Topic'',''TL_Merge''),else, web([''jar:file:///'',matlabroot,''/help/toolbox/simulink/help.jar!/slref/' lower(get_param(gcbh,'Blocktype')) '.html''], ''-helpbrowser''),end'])
      mask Display: plot([-0.05, 1.05, NaN, -0.05, 1.05],[.01, .01, NaN, .99, .99])
  RSFlipFlop : Subsystem  mask(TLMSR_V200_RSFlipFlop){dT=-1, QName=, QNName=}
      mask prompts: dT "SampleTime"; QName "Q OutName"; QNName "QN OutName"
      mask help: A flip flop. The 'R' input (reset) dominates the 'S' input (set).
      mask init:
      | % TL block lines
      | x1=[0 0 1 1 0];
      | y1=[1 0 0 1 1];
      | x2=[1 0];
      | y2=[.96 .96];
      | x3=[0 1];
      | y3=[.04 .04];
      | 
      | tl_act_sg_init_blk;
      mask Help:
      | <HTML>
      | <HEAD>
      | <META HTTP-EQUIV="Content-Type" CONTENT="text/html; charset=iso-8859-1">
      | <TITLE>test</TITLE>
      | </HEAD>
      | 
      | <B><FONT FACE="Arial"><P>Function:</P>
      | </B><P>The block provides the function of a RS-Flip-Flop with the reset input </FONT><FONT FACE="Courier New">R</FONT><FONT FACE="Arial"> dominating over the set input </FONT><FONT FACE="Courier New">S</FONT><FONT FACE="Arial">. An inverted output </FONT><FONT FACE="Courier New">/Q</FONT><FONT FACE="Arial"> is provided.</P>
      | </FONT>
      | <TABLE BORDER CELLSPACING=1 CELLPADDING=4 WIDTH=506>
      | <TR><TD WIDTH="25%" VALIGN="TOP">
      | <B><FONT FACE="Arial"><P ALIGN="CENTER">S</B></FONT></TD>
      | <TD WIDTH="25%" VALIGN="TOP">
      | <B><FONT FACE="Arial"><P ALIGN="CENTER">R</B></FONT></TD>
      | <TD WIDTH="25%" VALIGN="TOP">
      | <B><FONT FACE="Arial"><P ALIGN="CENTER">Q</B></FONT></TD>
      | <TD WIDTH="25%" VALIGN="TOP">
      | <B><FONT FACE="Arial"><P ALIGN="CENTER">/Q</B></FONT></TD>
      | </TR>
      | <TR><TD WIDTH="25%" VALIGN="TOP">
      | <FONT FACE="Arial"><P ALIGN="CENTER">0</FONT></TD>
      | <TD WIDTH="25%" VALIGN="TOP">
      | <FONT FACE="Arial"><P ALIGN="CENTER">0</FONT></TD>
      | <TD WIDTH="25%" VALIGN="TOP">
      | <FONT FACE="Arial"><P ALIGN="CENTER">Q(n-1)</FONT></TD>
      | <TD WIDTH="25%" VALIGN="TOP">
      | <FONT FACE="Arial"><P ALIGN="CENTER">/Q(n-1)</FONT></TD>
      | </TR>
      | <TR><TD WIDTH="25%" VALIGN="TOP">
      | <FONT FACE="Arial"><P ALIGN="CENTER">0</FONT></TD>
      | <TD WIDTH="25%" VALIGN="TOP">
      | <FONT FACE="Arial"><P ALIGN="CENTER">1</FONT></TD>
      | <TD WIDTH="25%" VALIGN="TOP">
      | <FONT FACE="Arial"><P ALIGN="CENTER">0</FONT></TD>
      | <TD WIDTH="25%" VALIGN="TOP">
      | <FONT FACE="Arial"><P ALIGN="CENTER">1</FONT></TD>
      | </TR>
      | <TR><TD WIDTH="25%" VALIGN="TOP">
      | <FONT FACE="Arial"><P ALIGN="CENTER">1</FONT></TD>
      | <TD WIDTH="25%" VALIGN="TOP">
      | <FONT FACE="Arial"><P ALIGN="CENTER">0</FONT></TD>
      | <TD WIDTH="25%" VALIGN="TOP">
      | <FONT FACE="Arial"><P ALIGN="CENTER">1</FONT></TD>
      | <TD WIDTH="25%" VALIGN="TOP">
      | <FONT FACE="Arial"><P ALIGN="CENTER">0</FONT></TD>
      | </TR>
      | <TR><TD WIDTH="25%" VALIGN="TOP">
      | <FONT FACE="Arial"><P ALIGN="CENTER">1</FONT></TD>
      | <TD WIDTH="25%" VALIGN="TOP">
      | <FONT FACE="Arial"><P ALIGN="CENTER">1</FONT></TD>
      | <TD WIDTH="25%" VALIGN="TOP">
      | <FONT FACE="Arial"><P ALIGN="CENTER">0</FONT></TD>
      | <TD WIDTH="25%" VALIGN="TOP">
      | <FONT FACE="Arial"><P ALIGN="CENTER">1</FONT></TD>
      | </TR>
      | </TABLE>
      | 
      | <FONT FACE="Arial">
      | <B><P>In-/Outputs:</P>
      | </B><U><P>S</P>
      | </U><P>The set input </FONT><FONT FACE="Courier New">S</FONT><FONT FACE="Arial"> on '1' will set the output </FONT><FONT FACE="Courier New">Q</FONT><FONT FACE="Arial"> if the reset input </FONT><FONT FACE="Courier New">R</FONT><FONT FACE="Arial"> is '0'.</P>
      | <U><P>R</P>
      | </U><P>The reset input </FONT><FONT FACE="Courier New">R</FONT><FONT FACE="Arial"> on '1' will reset the output </FONT><FONT FACE="Courier New">Q</FONT><FONT FACE="Arial">.</P>
      | <U><P>Q, /Q</P>
      | </U><P>The output </FONT><FONT FACE="Courier New">Q</FONT><FONT FACE="Arial"> shows the state of the internal memory. </FONT><FONT FACE="Courier New">/Q</FONT><FONT FACE="Arial"> contains the inverted state of </FONT><FONT FACE="Courier New">Q</FONT><FONT FACE="Arial">.</P></FONT>
      | </HTML>
      mask Display:
      | plot(x1,y1,x2,y2,x3,y3);
      | image(imread('RSFlipFlop.tif','tif'),[0.05,0.1,0.9,0.8])
  Terminator : Terminator
  VERSION_INFO : Subsystem  mask(VERSION_INFO_BLOCK){versinfo_data=struct('modname','DEMO_FAS/DEMO_FAS_Funktion/Limiter/Limiter_Function/Limiter_Enabled','version','1.1.1','date','18-Apr-2013','author','YVEDUHR','modtype',3,'variant',0,'remark',{{'~'}},'copyright',['Daimler AG'],'SGMLdescr','','prefix','','pfx_act',0,'ntselect',3,'asize',0), versinfo_string=Model: DEMO_FAS/DEMO_FAS_Funktion/Limiter/Limiter_Function/Limiter_Enabled\nVersion: 1.1.1\nDate: 18-Apr-2013\nAuthor: YVEDUHR\nModule: INTERNAL\n\nAll copyrights by Daimler AG}
      mask prompts: versinfo_data "Mask Parameter 1"; versinfo_string "Mask Parameter 2"
      mask help:
      | This is a Version Info Subsystem (empty)
      | All version Information is stored in Parameter "versinfo_data" and displayed
      settings: OpenFcn=edit_subsys_info('init')
      mask Display: disp(versinfo_string);
  VMax_kmh : Outport  InitialOutput=300
  Limiter_active_b : Outport  Port=2  InitialOutput=0
  wires:
  If/1 -> Limiter_Active/Action
  Logical Operator2/1 -> RSFlipFlop/2(R)
  RSFlipFlop/1(Q) -> If/2
  RSFlipFlop/2(NOT_Q) -> Terminator/1
  Limiter_b/1 -> Logical Operator2/1, Logical Operator1/1, EdgeRising/1(u)
  EdgeRising/1(y) -> RSFlipFlop/1(S)
  False/1(y) -> EdgeRising/3(IV)
  Logical Operator1/1 -> EdgeRising/2(R)
  Limiter_Active/2(Limiter_active_b) -> Bus Creator/2
  Limiter_Active/1(VMax_kmh) -> Bus Creator/1
  Limiter_Deactive/2(Limiter_active_b) -> Bus Creator1/2
  Limiter_Deactive/1(VMax_kmh) -> Bus Creator1/1
  Bus Creator/1 -> Merge/1
  Bus Creator1/1 -> Merge/2
  Merge/1 -> Bus Selector/1  "VMax_kmh"
  Bus Selector/1 -> VMax_kmh/1  "<VMax_kmh>"
  Bus Selector/2 -> Limiter_active_b/1  "<Limiter_active_b>"
  Accelaration_pedal_pc/1 -> If/1
  If/2 -> Limiter_Deactive/Action

== system DAS/DEMO_FAS/DEMO_FAS/Subsystem/DEMO_FAS/DEMO_FAS_Funktion/Limiter/Limiter_Function/Limiter_InitialSetValue ==
  V_Vehicle_kmh : Inport
  Trigger : TriggerPort
  Data Store Write : DataStoreWrite  Description=|  DataStoreName=DEMO_FAS_V_LimiterSetValue  mask(TL_DataStoreWrite){data={'date',735342.52783787041}}
      | Data Store Write block of dSPACE TargetLink.
      | Use this block to specify outputs to global variables within the production code application.
      settings: DeleteFcn=if exist('delete_tlblock','file')==2,delete_tlblock(gcbh);end  NameChangeFcn=if exist('rename_tlblock','file')==2,rename_tlblock(gcbh);end  OpenFcn=if exist('tl_open_blockdlg','file')==2,tl_open_blockdlg(gcbh);else,open_system(gcbh,'parameter');end
      mask Help: eval(['if exist(''tl_online_help'',''file'') == 2, tl_online_help(''Topic'',''TL_DataStoreWrite''),else, web([''jar:file:///'',matlabroot,''/help/toolbox/simulink/help.jar!/slref/' lower(get_param(gcbh,'Blocktype')) '.html''], ''-helpbrowser''),end'])
      mask Display: plot([-0.05, 1.05, NaN, -0.05, 1.05],[.01, .01, NaN, .99, .99])
  VERSION_INFO : Subsystem  mask(VERSION_INFO_BLOCK){versinfo_data=struct('modname','DEMO_FAS/DEMO_FAS_Funktion/Limiter/Limiter_Function/Limiter_InitialSetValue','version','1.1.1','date','18-Apr-2013','author','YVEDUHR','modtype',3,'variant',0,'remark',{{'~'}},'copyright',['Daimler AG'],'SGMLdescr','','prefix','','pfx_act',0,'ntselect',3,'asize',0), versinfo_string=Model: DEMO_FAS/DEMO_FAS_Funktion/Limiter/Limiter_Function/Limiter_InitialSetValue\nVersion: 1.1.1\nDate: 18-Apr-2013\nAuthor: YVEDUHR\nModule: INTERNAL\n\nAll copyrights by Daimler AG}
      mask prompts: versinfo_data "Mask Parameter 1"; versinfo_string "Mask Parameter 2"
      mask help:
      | This is a Version Info Subsystem (empty)
      | All version Information is stored in Parameter "versinfo_data" and displayed
      settings: OpenFcn=edit_subsys_info('init')
      mask Display: disp(versinfo_string);
  wires:
  V_Vehicle_kmh/1 -> Data Store Write/1
